simulink model "schema_di_controllo"  (R2024b)
settings: Solver=VariableStepAuto  StartTime=0.0  StopTime=0.1  RelTol=1e-3
values from neighbouring files (symbols this model uses):
  C = [1 0]    [G_s_linearizzata.m]    (also in progetto_carrello_soluzione.m)
  u_e = k*x_e1/tau(x_e1)    [G_s_linearizzata.m]    (also in progetto_carrello_soluzione.m = 20)
  x_e1 = theta_e_rad    [G_s_linearizzata.m]
libraries: cstblocks x1
settings Model: Creator=guidocarnevale  LastModifiedBy=tomma
settings RTWCC: GPUComputeCapability=3.5

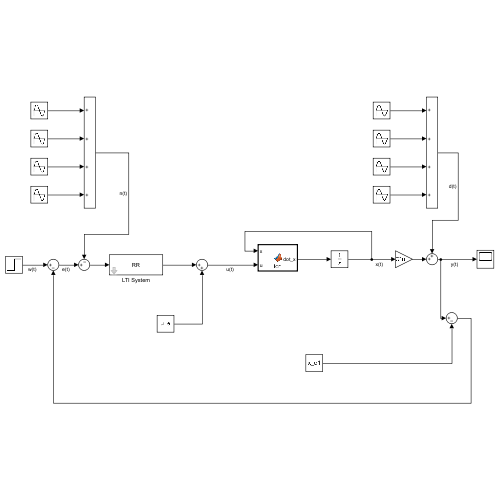
[thumbnail: Simulink's stored preview of the top-level diagram]
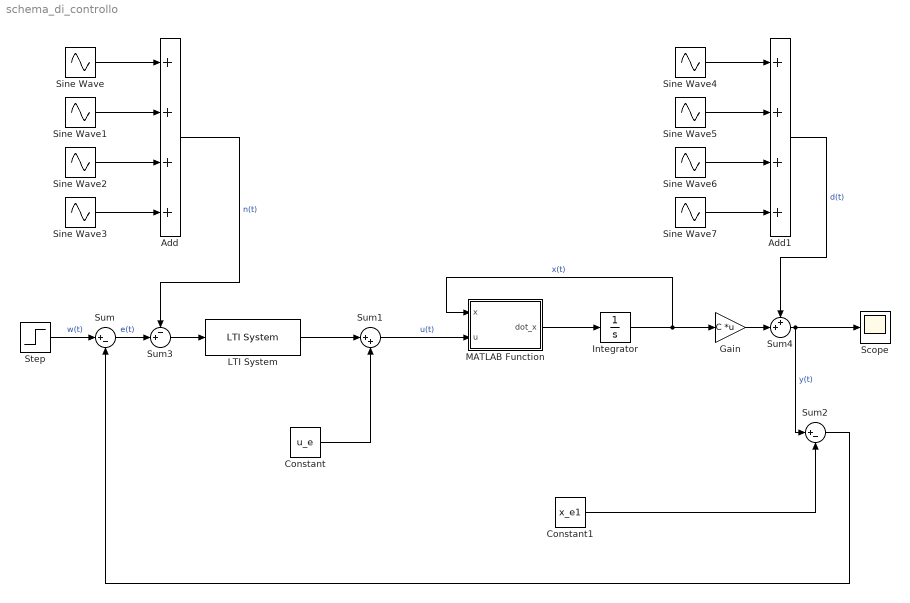
== system schema_di_controllo ==
  Add : Sum  Inputs=++++
  Add1 : Sum  Inputs=++++
  Constant : Constant  Value=u_e  VectorParams1D=off
  Constant1 : Constant  Value=x_e1
  Gain : Gain  Gain=C  Multiplication=Matrix(K*u)
  Integrator : Integrator
  LTI System : cstblocks/LTI System  sys=RR  IC=[]  PadeOrder=0
  MATLAB Function : MATLAB Function  TreatAsAtomicUnit=on
  Scope : Scope
  Sine Wave : Sin  Amplitude=0.2  Frequency=10^5  SampleTime=0
  Sine Wave1 : Sin  Amplitude=0.2  Frequency=2*10^5  SampleTime=0
  Sine Wave2 : Sin  Amplitude=0.2  Frequency=3*10^5  SampleTime=0
  Sine Wave3 : Sin  Amplitude=0.2  Frequency=4*10^5  SampleTime=0
  Sine Wave4 : Sin  Amplitude=0.2  Frequency=0.1  SampleTime=0
  Sine Wave5 : Sin  Amplitude=0.2  Frequency=2*0.1  SampleTime=0
  Sine Wave6 : Sin  Amplitude=0.2  Frequency=3*0.1  SampleTime=0
  Sine Wave7 : Sin  Amplitude=0.2  Frequency=4*0.1  SampleTime=0
  Step : Step  Time=0  SampleTime=0
  Sum : Sum  Inputs=|+-
  Sum1 : Sum  Inputs=|++
  Sum2 : Sum  Inputs=|+-
  Sum3 : Sum  Inputs=-+|
  Sum4 : Sum  Inputs=++|
  wires:
  MATLAB Function/1(dot_x) -> Integrator/1
  Integrator/1 -> MATLAB Function/1(x), Gain/1  "x(t)"
  Step/1 -> Sum/1  "w(t)"
  LTI System/1 -> Sum1/1
  Constant/1 -> Sum1/2
  Sum1/1 -> MATLAB Function/2(u)  "u(t)"
  Sum2/1 -> Sum/2
  Constant1/1 -> Sum2/2
  Sine Wave/1 -> Add/1
  Sine Wave1/1 -> Add/2
  Sine Wave2/1 -> Add/3
  Sine Wave3/1 -> Add/4
  Sine Wave7/1 -> Add1/4
  Sine Wave5/1 -> Add1/2
  Sine Wave6/1 -> Add1/3
  Sine Wave4/1 -> Add1/1
  Sum3/1 -> LTI System/1
  Add/1 -> Sum3/1  "n(t)"
  Sum/1 -> Sum3/2  "e(t)"
  Gain/1 -> Sum4/2
  Sum4/1 -> Sum2/1, Scope/1  "y(t)"
  Add1/1 -> Sum4/1  "d(t)"

== matlab function schema_di_controllo/MATLAB Function ==
  data: x input; u input; dot_x output
function dot_x = fcn(x,u)

k = 100; % elasticità del disco
beta = 0.6; % attrito viscoso
alpha = 30; % angolo in gradi tra i due alberi
J = 800; % momento di inerzia della tavola

alpha_rad = deg2rad(alpha);

tau = @(theta) cos(alpha_rad)/(1-(sin(alpha_rad)*cos(theta))^2);

dot_x = zeros(2,1);

dot_x(1) = x(2);

dot_x(2) = tau(x(1))*u/J-(beta*x(2))/J-k*x(1)/J;
